simulink model "forced_msd"  (Simulink 7.8)
settings: Solver=ode4  StartTime=0.0  StopTime=time_span  RelTol=1e-3
undefined symbols (not defined in the file or in its folder): input_set, outstr, samp_time, step_size
settings Model: Creator=Kourosh Danai  LastModifiedBy=Bill
settings DataIOCC: TimeSaveName=t  OutputSaveName=y
settings DebuggingCC: AlgebraicLoopMsg=none  FcnCallInpInsideContextMsg=Use local settings  StrictBusMsg=Warning
settings SFSimCC: SimParseCustomCode=off

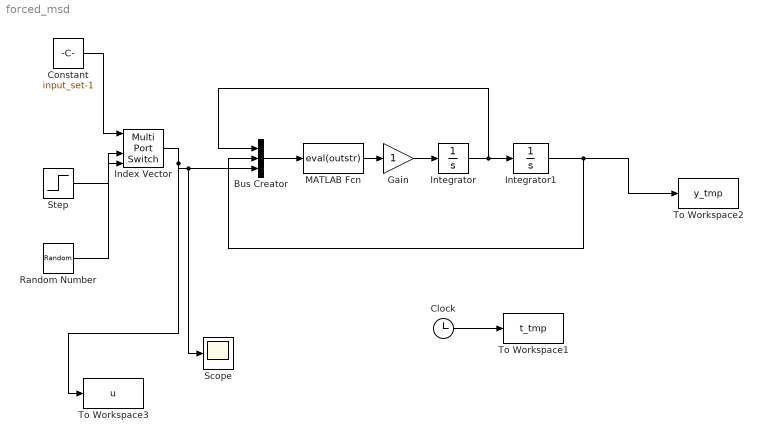
== system forced_msd ==
  Bus Creator : BusCreator  Inputs=3
  Clock : Clock
  Constant : Constant  Value=input_set-1
  Gain : Gain
  Index Vector : MultiPortSwitch  DataPortOrder=Zero-based contiguous  zeroidx=on
  Integrator : Integrator
  Integrator1 : Integrator
  MATLAB Fcn : MATLABFcn  MATLABFcn=eval(outstr)
  Random Number : RandomNumber  SampleTime=0
  Scope : Scope
  Step : Step  Time=0  After=step_size  SampleTime=samp_time
  To Workspace1 : ToWorkspace  VariableName=t_tmp  SampleTime=-1  SaveFormat=Array
  To Workspace2 : ToWorkspace  VariableName=y_tmp  SampleTime=-1  SaveFormat=Array
  To Workspace3 : ToWorkspace  VariableName=u  SampleTime=-1  SaveFormat=Array
  wires:
  Integrator/1 -> Integrator1/1, Bus Creator/1
  Bus Creator/1 -> MATLAB Fcn/1
  MATLAB Fcn/1 -> Gain/1
  Gain/1 -> Integrator/1
  Step/1 -> Index Vector/3
  Constant/1 -> Index Vector/1
  Index Vector/1 -> Scope/1, Bus Creator/3, To Workspace3/1
  Random Number/1 -> Index Vector/4
  Integrator1/1 -> Bus Creator/2, To Workspace2/1
  Clock/1 -> To Workspace1/1
